simulink model "chap9_8sim"  (Simulink 5.0)
settings: Solver=ode45  StartTime=0.0  StopTime=30  RelTol=1e-3
settings Model: LastModifiedBy=Administrator

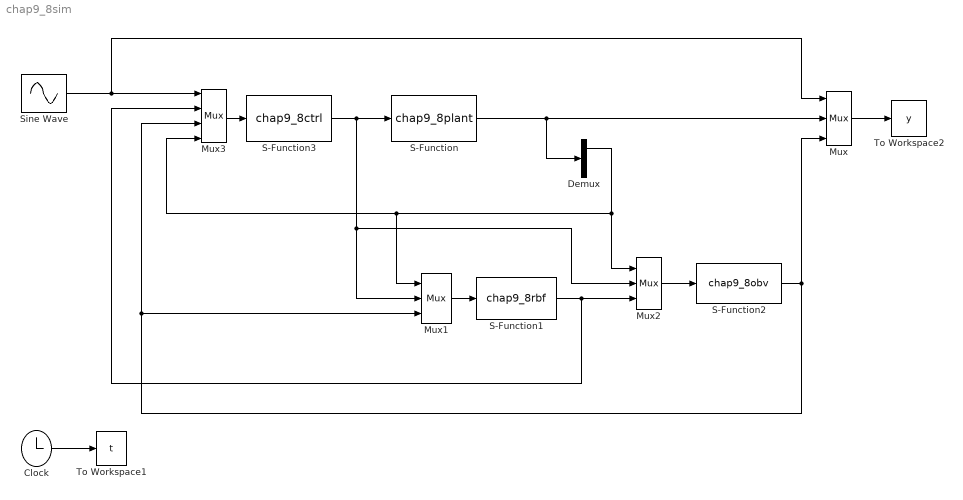
== system chap9_8sim ==
  Clock : Clock
      settings: Decimation=10
  Demux : Demux  Outputs=2
  Mux : Mux  Inputs=3
  Mux1 : Mux  Inputs=3
  Mux2 : Mux  Inputs=3
  Mux3 : Mux
  S-Function : S-Function  FunctionName=chap9_8plant
  S-Function1 : S-Function  FunctionName=chap9_8rbf
  S-Function2 : S-Function  FunctionName=chap9_8obv
  S-Function3 : S-Function  FunctionName=chap9_8ctrl
  Sine Wave : Sin  SampleTime=0
  To Workspace1 : ToWorkspace  VariableName=t  SampleTime=-1  SaveFormat=Array
  To Workspace2 : ToWorkspace  VariableName=y  SampleTime=-1  SaveFormat=Array
  wires:
  Clock/1 -> To Workspace1/1
  Mux/1 -> To Workspace2/1
  S-Function2/1 -> Mux1/3, Mux3/3, Mux/3
  Mux1/1 -> S-Function1/1
  Mux2/1 -> S-Function2/1
  S-Function1/1 -> Mux2/3, Mux3/2
  S-Function/1 -> Demux/1, Mux/2
  Demux/1 -> Mux2/1, Mux1/1, Mux3/4
  S-Function3/1 -> S-Function/1, Mux1/2, Mux2/2
  Sine Wave/1 -> Mux3/1, Mux/1
  Mux3/1 -> S-Function3/1
